simulink model "Control_software_v1_1"  (R2017a)
settings: Solver=FixedStepDiscrete  StartTime=0.0  StopTime=inf  FixedStep=Ts_main  RelTol=1e-3  EnableMultiTasking=on
InitFcn:
  | clc
  | eval('ContrPrm_v1_1')
model workspace (MAT data in the model file):
  JoyW_sat = 10
values from neighbouring files (symbols this model uses):
  Afilt_Winch = (Amatr_Winch-L_Winch*Cmatr_Winch)    [ContrPrm_v1_1.m]
  AOsat = 10    [ContrPrm_v1_1.m]
  Bfilt_Winch = [L_Winch Bmatr_Winch]    [ContrPrm_v1_1.m]
  Cfilt_Winch = eye(2)    [ContrPrm_v1_1.m]
  Dfilt_Winch = zeros(2)    [ContrPrm_v1_1.m]
  JoyS_gain = 5    [ContrPrm_v1_1.m]
  JoyS_ofst = -2.5    [ContrPrm_v1_1.m]
  JoyS_sat = 9.2    [ContrPrm_v1_1.m]
  JoyW_gain = -5    [ContrPrm_v1_1.m]
  JoyW_ofst = -2.5    [ContrPrm_v1_1.m]
  KspdWinch = 1    [ContrPrm_v1_1.m]
  NPotSpdEst = 3    [ContrPrm_v1_1.m]
  Pot_gain = PotMax/5    (= 0.08)    [ContrPrm_v1_1.m]
  Pot_max = PotMax    (= 0.4)    [ContrPrm_v1_1.m]
  Pot_min = 0    [ContrPrm_v1_1.m]
  Pot_ofst = -0.0558    [ContrPrm_v1_1.m]
  Ts_1ms = 1e-3    (= 0.001)    [ContrPrm_v1_1.m]
  Ts_1s = 1    [ContrPrm_v1_1.m]
  WinchDrumRad = 0.1    [ContrPrm_v1_1.m]
  WinchMotPosAIgain = WinchRevMax/WinchVoltMax*rev2rad    (= 76)    [ContrPrm_v1_1.m]
  WinchMotTorqueMax = 13    [ContrPrm_v1_1.m]
  WinchRefSpdSup = 15/WinchDrumRad    (= 150)    [ContrPrm_v1_1.m]
  WinchTravelMin_m = -2    [ContrPrm_v1_1.m]
  WinchVoltMax = 10    [ContrPrm_v1_1.m]
  x0_Winch = [0;0]    [ContrPrm_v1_1.m]
undefined symbols (not defined in the file or in its folder): C, datevec, JoyFiltDen, JoyFiltNum, PotPosFiltDen, PotPosFiltNum, WinchPosFiltDen, WinchPosFiltNum, WinchSpdEstFiltDen, WinchSpdEstFiltNum
libraries: xpcnilib x6, slrtlib x6, xpcseriallib x4, simulink x4, speedgoatlib_IO751 x3, etargetslib x2, xpcwalltimelib x1
(part 1 of 2)
settings Model: sg_rtwmakecfg_data=_sg_netxLib_MSVC140_  SimulationMode=external  Creator=Philip Hu  LastModifiedBy=admin
settings SolverCC: EnableConcurrentExecution=on
settings DataIOCC: SaveFormat=Array  SignalLoggingSaveFormat=ModelDataLogs  SaveOutput=off  SignalLogging=off  SaveTime=off
settings OptimizationCC: BlockReduction=off  OptimizeBlockIOStorage=off  BufferReuse=off  GlobalBufferReuse=off  ExpressionFolding=off  ExpressionDepthLimit=2147483647  LocalBlockOutputs=off  LifeSpan=inf
settings DebuggingCC: SolverPrmCheckMsg=warning  FcnCallInpInsideContextMsg=warning  StateNameClashWarn=warning  SFUnexpectedBacktrackingDiag=warning  SFNoUnconditionalDefaultTransitionDiag=warning  SFExecutionAtInitializationDiag=none
settings HardwareCC: ProdBitPerPointer=32  ProdBitPerSizeT=32  ProdBitPerPtrDiffT=32  ProdLargestAtomicFloat=None  ProdWordSize=32  ProdLongLongMode=on  ProdHWDeviceType=Generic->32-bit x86 compatible
settings ModelReferenceCC: PropagateSignalLabelsOutOfModel=off
settings SFSimCC: SimParseCustomCode=off
settings RTWCC: SystemTargetFile=slrt.tlc  TemplateMakefile=slrt_default_tmf  Description=Simulink Real-Time  RTWCompilerOptimization=on
settings SimulinkRealTimeCC: GeneratePreprocessorConditionals=Disable all  RL32ObjectName=AWE  xPCModelTimeoutSecs=20
settings ConfigComp: CovMetricSettings=dw  CovHtmlReporting=on  CovSaveCumulativeToWorkspaceVar=on  CovSaveSingleToWorkspaceVar=on  CovExternalEMLEnable=off  CovSFcnEnable=off

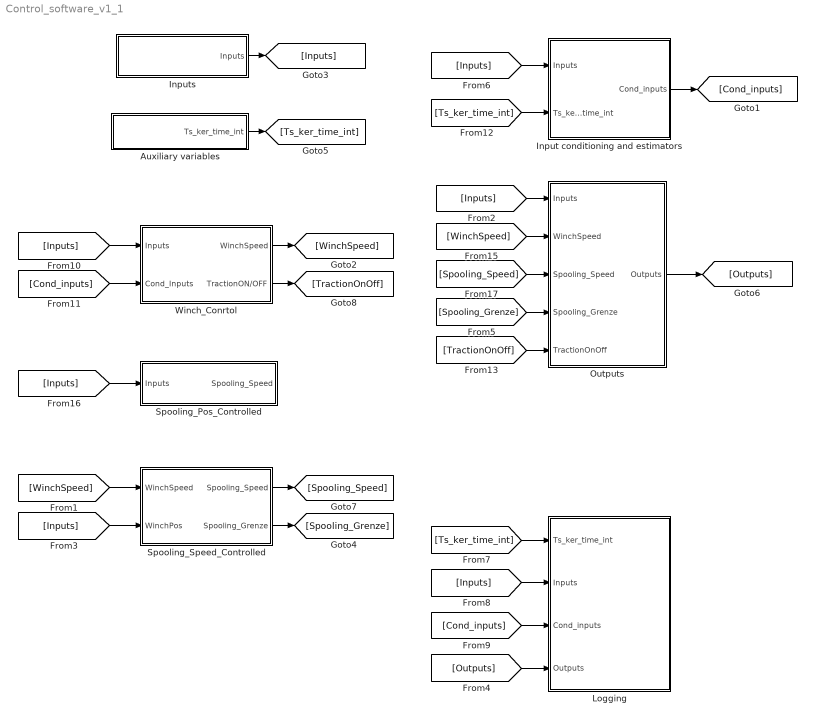
== system Control_software_v1_1 ==
  Auxiliary variables : Subsystem
  Input conditioning and estimators : Subsystem
  Inputs : Subsystem
  Logging : Subsystem
  Outputs : Subsystem
  Spooling_Pos_Controlled : Subsystem
  Spooling_Speed_Controlled : Subsystem
  Winch_Conrtol : Subsystem
  wires:
  Auxiliary variables/1(Ts_ker_time_int) -> [Ts_ker_time_int]
  [Ts_ker_time_int] -> Logging/1(Ts_ker_time_int)
  Outputs/1(Outputs) -> [Outputs]
  [Cond_inputs] -> Logging/3(Cond_inputs)
  Inputs/1(Inputs) -> [Inputs]
  Input conditioning and estimators/1(Cond_inputs) -> [Cond_inputs]
  [Outputs] -> Logging/4(Outputs)
  [Inputs] -> Input conditioning and estimators/1(Inputs)
  [Inputs] -> Logging/2(Inputs)
  [Ts_ker_time_int] -> Input conditioning and estimators/2(Ts_ker_time_int)
  [Inputs] -> Outputs/1(Inputs)
  [Inputs] -> Winch_Conrtol/1(Inputs)
  [Cond_inputs] -> Winch_Conrtol/2(Cond_Inputs)
  Winch_Conrtol/1(WinchSpeed) -> [WinchSpeed]
  [WinchSpeed] -> Outputs/2(WinchSpeed)
  [Inputs] -> Spooling_Pos_Controlled/1(Inputs)
  [Spooling_Speed] -> Outputs/3(Spooling_Speed)
  [WinchSpeed] -> Spooling_Speed_Controlled/1(WinchSpeed)
  [Inputs] -> Spooling_Speed_Controlled/2(WinchPos)
  Spooling_Speed_Controlled/1(Spooling_Speed) -> [Spooling_Speed]
  Spooling_Speed_Controlled/2(Spooling_Grenze) -> [Spooling_Grenze]
  [Spooling_Grenze] -> Outputs/4(Spooling_Grenze)
  Winch_Conrtol/2(TractionON/OFF) -> [TractionOnOff]
  [TractionOnOff] -> Outputs/5(TractionOnOff)

== system Control_software_v1_1/Auxiliary variables ==
  Constat : Constant  Value=Ts_1s  SampleTime=Ts_1s
  Sum : Sum  Inputs=|++
  Unit Delay : UnitDelay  SampleTime=-1
  Ts_ker_time_int : Outport
  wires:
  Constat/1 -> Sum/1
  Sum/1 -> Ts_ker_time_int/1, Unit Delay/1
  Unit Delay/1 -> Sum/2

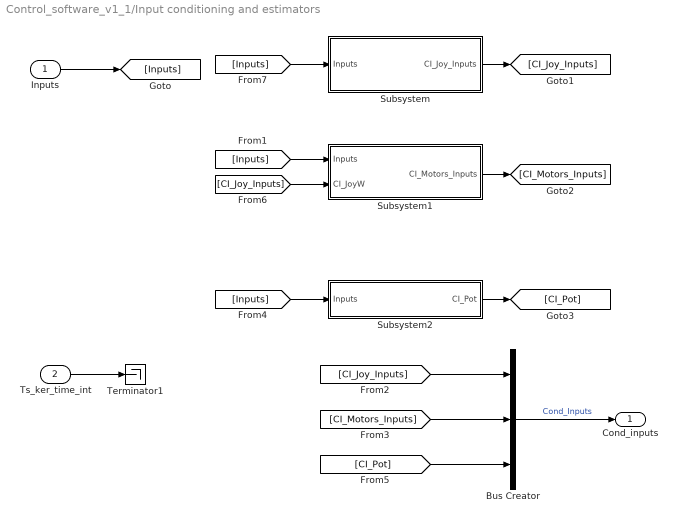
== system Control_software_v1_1/Input conditioning and estimators ==
  Inputs : Inport
  Ts_ker_time_int : Inport  Port=2
  Bus Creator : BusCreator  Inputs=3
  Subsystem : Subsystem
  Subsystem1 : Subsystem
  Subsystem2 : Subsystem
  Terminator1 : Terminator
  Cond_inputs : Outport
  wires:
  Inputs/1 -> [Inputs]
  Ts_ker_time_int/1 -> Terminator1/1
  [Inputs] -> Subsystem/1(Inputs)
  Subsystem/1(CI_Joy_Inputs) -> [CI_Joy_Inputs]
  Bus Creator/1 -> Cond_inputs/1  "Cond_Inputs"
  [Inputs] -> Subsystem1/1(Inputs)
  Subsystem1/1(CI_Motors_Inputs) -> [CI_Motors_Inputs]
  [Inputs] -> Subsystem2/1(Inputs)
  Subsystem2/1(CI_Pot) -> [CI_Pot]
  [CI_Pot] -> Bus Creator/3
  [CI_Motors_Inputs] -> Bus Creator/2
  [CI_Joy_Inputs] -> Bus Creator/1
  [CI_Joy_Inputs] -> Subsystem1/2(CI_JoyW)

== system Control_software_v1_1/Inputs ==
  Analog Inputs : Subsystem
  Bus Creator2 : BusCreator  Inputs=5
  Digital Inputs : Subsystem
  RS232_read : Subsystem
  Inputs : Outport
  wires:
  Analog Inputs/1(Analog_inputs) -> Bus Creator2/1
  Digital Inputs/1(DgInputs) -> Bus Creator2/2
  Bus Creator2/1 -> Inputs/1
  RS232_read/2(GPS_data) -> Bus Creator2/4
  RS232_read/1(IMU_data) -> Bus Creator2/3
  RS232_read/3(GU_Yaw) -> Bus Creator2/5

== system Control_software_v1_1/Logging ==
  Ts_ker_time_int : Inport
  Inputs : Inport  Port=2
  Cond_inputs : Inport  Port=3
  Outputs : Inport  Port=4
  Bus Creator1 : BusCreator  Inputs=2
  Data Type Conversion1 : DataTypeConversion  OutDataTypeStr=double
  Log_conditioning : Subsystem
  MavLink_log : slrtlib/Displays and Logging/Scope   scopeno=1  scopetype=File  autostart=on  viewmode=Graphical redraw  formatstr='%15.6f'  grid=on  ylimits=[0,0]  nosamples=1000  noprepostsamples=0  interleave=1  triggermode=FreeRun  triggersignal=1  trigsignalfromport=off  triggerlevel=0.0  triggerslope=Either  triggerscope=1  triggersample=0  filename=Var_MVLK.dat  mode=Lazy  writesize=512  autorestart=on  dynamicfilemode=off  maxwritefilesize=512*1024^2
  TS100_log : slrtlib/Displays and Logging/Scope   scopeno=3  scopetype=File  autostart=on  viewmode=Graphical redraw  formatstr='%15.6f'  grid=on  ylimits=[0,0]  nosamples=1000  noprepostsamples=0  interleave=1  triggermode=FreeRun  triggersignal=1  trigsignalfromport=off  triggerlevel=0.0  triggerslope=Either  triggerscope=1  triggersample=0  filename=Var_100.dat  mode=Commit  writesize=512  autorestart=on  dynamicfilemode=off  maxwritefilesize=512*1024^2
  TS1_log : slrtlib/Displays and Logging/Scope   scopeno=2  scopetype=File  autostart=on  viewmode=Graphical redraw  formatstr='%15.6f'  grid=on  ylimits=[0,0]  nosamples=1000  noprepostsamples=0  interleave=1  triggermode=FreeRun  triggersignal=1  trigsignalfromport=off  triggerlevel=0.0  triggerslope=Either  triggerscope=1  triggersample=0  filename=Var_1.dat  mode=Commit  writesize=512  autorestart=on  dynamicfilemode=off  maxwritefilesize=512*1024^2
  Time_Scope_trigger : Subsystem
  Time_log : slrtlib/Displays and Logging/Scope   scopeno=4  scopetype=File  autostart=on  viewmode=Graphical sliding  formatstr='%15.6f'  grid=off  ylimits=[0,0]  nosamples=10  noprepostsamples=0  interleave=1  triggermode=Signal triggering  triggersignal=2  trigsignalfromport=off  triggerlevel=0.5  triggerslope=Either  triggerscope=1  triggersample=0  filename=Var_Time.dat  mode=Commit  writesize=512  autorestart=off  dynamicfilemode=off  maxwritefilesize=512*1024^2
  Wall Time 1 : xpcwalltimelib/Wall Time   TimeFormat=Date  EpochSource=MATLAB  EpochVector=datevec('01/01/1970')  InputTrigger=off  SampleTime=Ts_1s
  wires:
  Log_conditioning/2(T100_log) -> TS100_log/1
  Bus Creator1/1 -> Time_log/1  "Date_time"
  Time_Scope_trigger/1(Trigger_time) -> Bus Creator1/2
  Ts_ker_time_int/1 -> Time_Scope_trigger/1(In1)
  Outputs/1 -> Log_conditioning/3(Outputs)
  Cond_inputs/1 -> Log_conditioning/2(Cond_inputs)
  Inputs/1 -> Log_conditioning/1(Inputs)
  Log_conditioning/1(MaVLink_log) -> MavLink_log/1
  Log_conditioning/3(T1_log) -> TS1_log/1
  Wall Time 1/1 -> Data Type Conversion1/1
  Data Type Conversion1/1 -> Bus Creator1/1

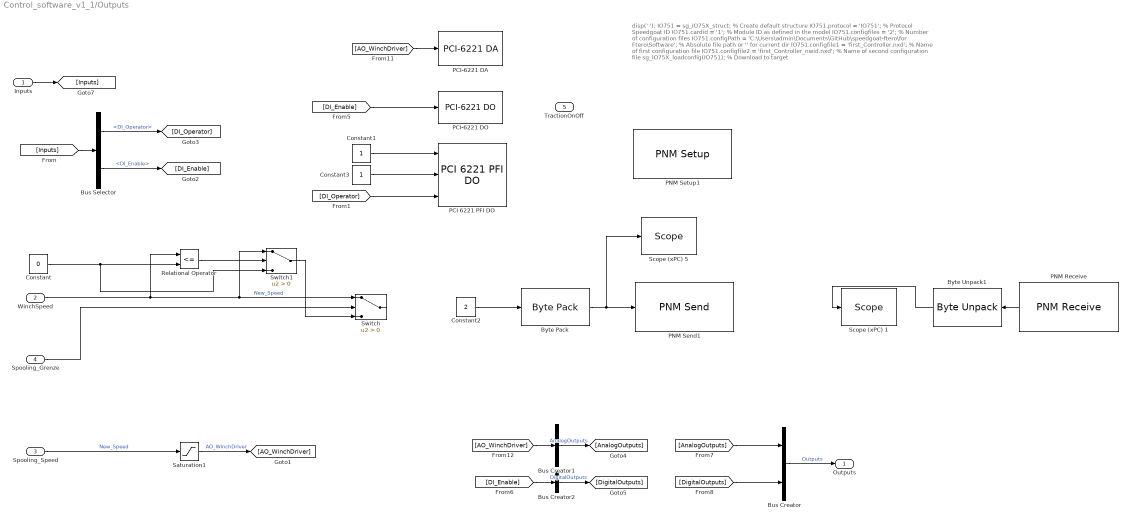
== system Control_software_v1_1/Outputs ==
  note: disp(' ');
      |     IO751 = sg_IO75X_struct;				 											% Create default structure
      |
      |     IO751.protocol = 'IO751';				 											% Protocol Speedgoat ID
      |     IO751.cardid = '1';						 											% Module ID as defined in the model
      |     IO751.configfiles = '2';					 											% Number of configuration files
      |     IO751.configPath = 'C:\Users\admin\Documents\GitHub\speedgoat-ftero\for Ftero\Software';	 % Absolute file path or '' for current dir
      |     IO751.configfile1 = 'first_Controller.nxd';	 											% Name of first configuration file
      |     IO751.configfile2 = 'first_Controller_nwid.nxd'; 											% Name of second configuration file
      |
      |     sg_IO75X_loadconfig(IO751);														% Download to target
  Inputs : Inport
  WinchSpeed : Inport  Port=2
  Spooling_Speed : Inport  Port=3
  Spooling_Grenze : Inport  Port=4
  TractionOnOff : Inport  Port=5
  Bus Creator : BusCreator  Inputs=2
  Bus Creator1 : BusCreator  Inputs=1
  Bus Creator2 : BusCreator  Inputs=1
  Bus Selector : BusSelector  OutputSignals=DgInputs.DI_Operator,DgInputs.DI_Enable
  Byte Pack : etargetslib/Byte Pack  datatypes={'uint8'}  byteAlign=1
  Byte Unpack1 : etargetslib/Byte Unpack  dimensions={1}  datatypes={'uint8'}  byteAlign=1
  Constant : Constant  Value=0
  Constant1 : Constant
  Constant2 : Constant  Value=2  OutDataTypeStr=uint8
  Constant3 : Constant
  "PCI 6221 PFI DO " : xpcnilib/Digital Output/M Series/PCI 6221 PFI DO   channel=[0 2 3]  reset=[0]  initial=[1 1 0]  sampleTime=Ts_1ms  slot=-1
      settings: SourceProductName=Simulink Real-Time  SourceProductBaseCode=XP
  PCI-6221 DA : xpcnilib/D//A/M Series/PCI-6221 DA  channel=[2]  reset=[1]  initValue=[0]  sampletime=Ts_1ms  slot=-1
      settings: SourceProductName=Simulink Real-Time  SourceProductBaseCode=XP
  PCI-6221 DO : xpcnilib/Digital Output/M Series/PCI-6221 DO  channel=[6]  reset=[0]  initValue=[0]  sampletime=Ts_1ms  slot=-1
      settings: SourceProductName=Simulink Real-Time  SourceProductBaseCode=XP
  PNM Receive : speedgoatlib_IO751/PNM Receive  id=1  portType=1 port with n element vector of type UINT8  inputOutput=1  sampleTime=0.001
  PNM Send1 : speedgoatlib_IO751/PNM Send  id=1  portType=1 port with n element vector of type UINT8  inputOutput=1  sampleTime=0.001
  PNM Setup1 : speedgoatlib_IO751/PNM Setup  id=1  driveLetter=C:  configurationMode=Configuration file  mode=Polling mode  sampleTime=0.001  pciSlot=-1  quantityOfAcyclicObjects=0
  Relational Operator : RelationalOperator  Operator=<=  OutDataTypeStr=boolean  RndMeth=Simplest
  Saturation1 : Saturate  UpperLimit=AOsat  LowerLimit=-AOsat
  Scope (xPC) 1 : slrtlib/Displays and Logging/Scope   scopeno=7  scopetype=Target  autostart=on  viewmode=Numerical  formatstr='%15.6f'  grid=on  ylimits=[0,0]  nosamples=3  noprepostsamples=0  interleave=1  triggermode=FreeRun  triggersignal=1  trigsignalfromport=off  triggerlevel=0.0  triggerslope=Either  triggerscope=1  triggersample=0  filename=data.dat  mode=Lazy  writesize=512  autorestart=off  dynamicfilemode=off  maxwritefilesize=512*1024^2
  Scope (xPC) 5 : slrtlib/Displays and Logging/Scope   scopeno=5  scopetype=Target  autostart=on  viewmode=Numerical  formatstr='%15.6f'  grid=on  ylimits=[0,0]  nosamples=3  noprepostsamples=0  interleave=1  triggermode=FreeRun  triggersignal=1  trigsignalfromport=off  triggerlevel=0.0  triggerslope=Either  triggerscope=1  triggersample=0  filename=data.dat  mode=Lazy  writesize=512  autorestart=off  dynamicfilemode=off  maxwritefilesize=512*1024^2
  Switch : Switch  Criteria=u2 > Threshold  OutDataTypeStr=uint8
  Switch1 : Switch  Criteria=u2 > Threshold
  Outputs : Outport
  wires:
  Inputs/1 -> [Inputs]
  [Inputs] -> Bus Selector/1
  Bus Creator/1 -> Outputs/1  "Outputs"
  [AnalogOutputs] -> Bus Creator/1
  [DigitalOutputs] -> Bus Creator/2
  Bus Selector/1 -> [DI_Operator]  "<DI_Operator>"
  Bus Creator1/1 -> [AnalogOutputs]  "AnalogOutputs"
  Bus Creator2/1 -> [DigitalOutputs]  "DigitalOutputs"
  Constant3/1 -> "PCI 6221 PFI DO "/2
  [AO_WinchDriver] -> PCI-6221 DA/1
  [AO_WinchDriver] -> Bus Creator1/1
  [DI_Enable] -> Bus Creator2/1
  [DI_Enable] -> PCI-6221 DO/1
  Bus Selector/2 -> [DI_Enable]  "<DI_Enable>"
  [DI_Operator] -> "PCI 6221 PFI DO "/3
  Constant1/1 -> "PCI 6221 PFI DO "/1
  Spooling_Speed/1 -> Saturation1/1  "New_Speed"
  WinchSpeed/1 -> Relational Operator/1, Switch1/1, Switch/1  "New_Speed"
  Spooling_Grenze/1 -> Switch/2
  Constant/1 -> Switch1/3, Relational Operator/2
  Relational Operator/1 -> Switch1/2
  Switch1/1 -> Switch/3
  Saturation1/1 -> [AO_WinchDriver]  "AO_WinchDriver"
  Byte Pack/1 -> Scope (xPC) 5/1, PNM Send1/1
  PNM Receive/1 -> Byte Unpack1/1
  Byte Unpack1/1 -> Scope (xPC) 1/1
  Constant2/1 -> Byte Pack/1

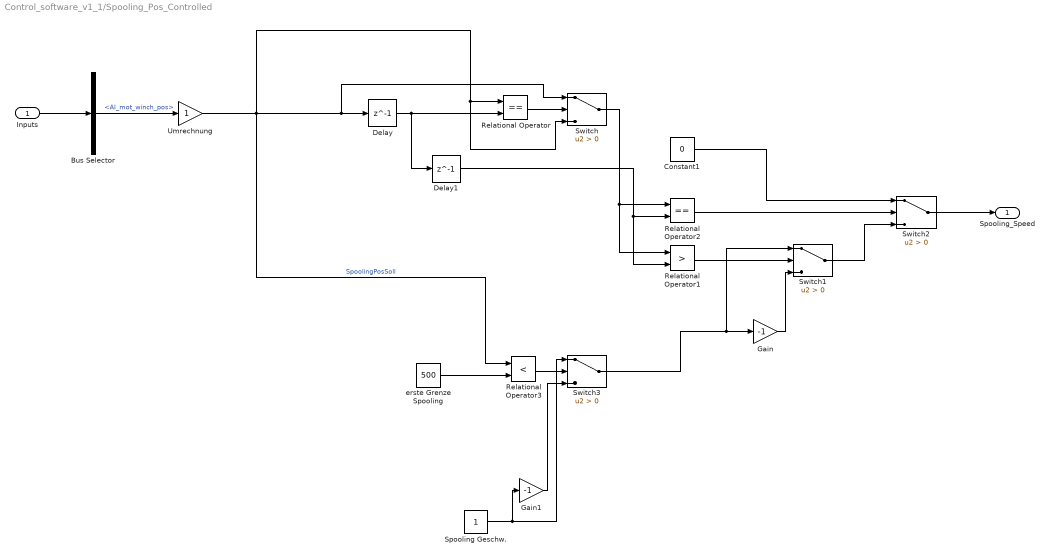
== system Control_software_v1_1/Spooling_Pos_Controlled ==
  Inputs : Inport
  Bus Selector : BusSelector  OutputSignals=Analog_inputs.AI_mot_winch_pos
  Constant1 : Constant  Value=0
  Delay : Delay  DelayLength=1  InitialCondition=0
  Delay1 : Delay  DelayLength=1  InitialCondition=0
  Gain : Gain  Gain=-1
  Gain1 : Gain  Gain=-1
  Relational Operator : RelationalOperator  Operator===  OutDataTypeStr=boolean  RndMeth=Simplest
  Relational Operator1 : RelationalOperator  Operator=>  OutDataTypeStr=boolean  RndMeth=Simplest
  Relational Operator2 : RelationalOperator  Operator===  OutDataTypeStr=boolean  RndMeth=Simplest
  Relational Operator3 : RelationalOperator  Operator=<  OutDataTypeStr=boolean  RndMeth=Simplest
  Spooling Geschw. : Constant
  Switch{,1..3} (4 alike) : Switch  Criteria=u2 > Threshold
  Umrechnung : Gain
  erste Grenze Spooling : Constant  Value=500
  Spooling_Speed : Outport
  wires:
  Inputs/1 -> Bus Selector/1
  Bus Selector/1 -> Umrechnung/1  "<AI_mot_winch_pos>"
  Umrechnung/1 -> Switch/3, Relational Operator/1, Relational Operator3/1, Switch/1, Delay/1  "SpoolingPosSoll"
  Relational Operator/1 -> Switch/2
  Switch/1 -> Relational Operator2/1, Relational Operator1/1
  Delay/1 -> Delay1/1, Relational Operator/2
  Relational Operator1/1 -> Switch1/2
  Constant1/1 -> Switch2/1
  Relational Operator2/1 -> Switch2/2
  Delay1/1 -> Relational Operator2/2, Relational Operator1/2
  Switch1/1 -> Switch2/3
  Gain/1 -> Switch1/3
  Relational Operator3/1 -> Switch3/2
  erste Grenze Spooling/1 -> Relational Operator3/2
  Switch3/1 -> Switch1/1, Gain/1
  Spooling Geschw./1 -> Gain1/1, Switch3/1
  Gain1/1 -> Switch3/3
  Switch2/1 -> Spooling_Speed/1

== system Control_software_v1_1/Spooling_Speed_Controlled ==
  WinchSpeed : Inport
  WinchPos : Inport  Port=2
  Bus Selector : BusSelector  OutputSignals=Analog_inputs.AI_mot_winch_pos
  Gain : Gain  Gain=-1
  Gain1 : Gain  Gain=2
  Relational Operator : RelationalOperator  Operator=<  OutDataTypeStr=boolean  RndMeth=Simplest
  Relational Operator1 : RelationalOperator  Operator=<  OutDataTypeStr=boolean  RndMeth=Simplest
  Spooling Grenze : Constant  Value=500
  Switch : Switch  Criteria=u2 > Threshold
  Umrechnung : Gain  Gain=0.01
  Umrechnung1 : Gain  Gain=0.1
  Spooling_Speed : Outport
  Spooling_Grenze : Outport  Port=2
  wires:
  WinchPos/1 -> Bus Selector/1
  Bus Selector/1 -> Umrechnung/1  "<AI_mot_winch_pos>"
  WinchSpeed/1 -> Umrechnung1/1
  Umrechnung/1 -> Relational Operator1/1, Relational Operator/1  "SpoolingPosSoll"
  Spooling Grenze/1 -> Gain1/1, Relational Operator/2
  Umrechnung1/1 -> Gain/1, Switch/1
  Gain/1 -> Switch/3
  Gain1/1 -> Relational Operator1/2
  Relational Operator/1 -> Switch/2
  Relational Operator1/1 -> Spooling_Grenze/1
  Switch/1 -> Spooling_Speed/1

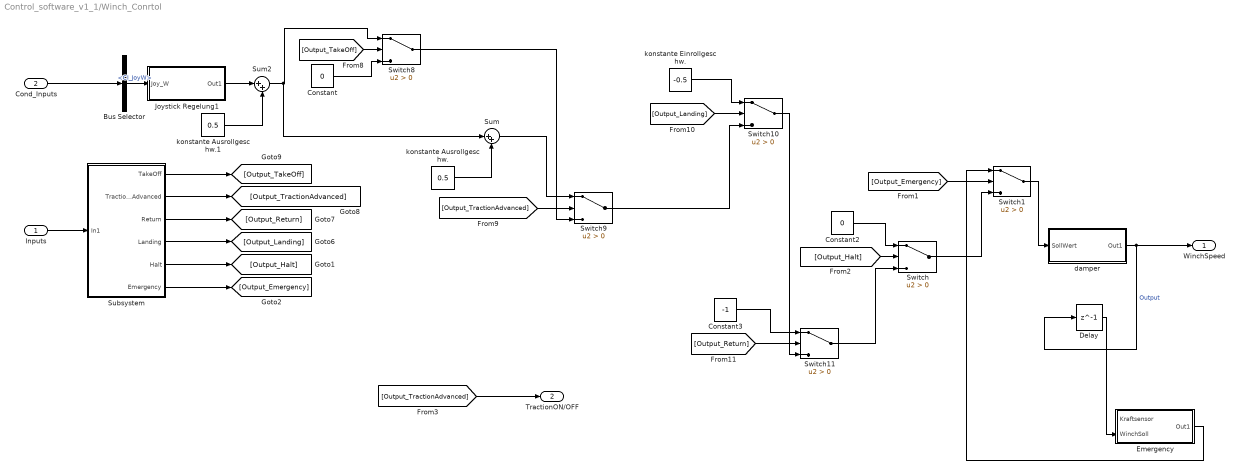
== system Control_software_v1_1/Winch_Conrtol ==
  Inputs : Inport
  Cond_Inputs : Inport  Port=2
  Bus Selector : BusSelector  OutputSignals=CI_Joy_Inputs.CI_JoyW
  Constant : Constant  Value=0
  Constant2 : Constant  Value=0
  Constant3 : Constant  Value=-1
  Delay : Delay  DelayLength=1  InitialCondition=0
  Emergency : Subsystem
  Joystick Regelung1 : Subsystem
  Subsystem : Subsystem
  Sum : Sum  Inputs=|++
  Sum2 : Sum  Inputs=|++
  Switch{,1,8..11} (6 alike) : Switch  Criteria=u2 > Threshold
  damper : Subsystem
  konstante Ausrollgeschw. : Constant  Value=0.5
  konstante Ausrollgeschw.1 : Constant  Value=0.5
  konstante Einrollgeschw. : Constant  Value=-0.5
  WinchSpeed : Outport
  TractionON/OFF : Outport  Port=2
  wires:
  Inputs/1 -> Subsystem/1(In1)
  [Output_TakeOff] -> Switch8/2
  [Output_TractionAdvanced] -> Switch9/2
  konstante Einrollgeschw./1 -> Switch10/1
  Switch10/1 -> Switch11/3
  [Output_Return] -> Switch11/2
  Subsystem/1(TakeOff) -> [Output_TakeOff]
  Subsystem/2(TractionAdvanced) -> [Output_TractionAdvanced]
  Subsystem/3(Return) -> [Output_Return]
  Subsystem/4(Landing) -> [Output_Landing]
  [Output_Landing] -> Switch10/2
  damper/1(Out1) -> WinchSpeed/1, Delay/1  "Output"
  Constant/1 -> Switch8/3
  Cond_Inputs/1 -> Bus Selector/1
  [Output_Halt] -> Switch/2
  [Output_Emergency] -> Switch1/2
  Constant2/1 -> Switch/1
  Switch11/1 -> Switch/3
  Switch/1 -> Switch1/3
  Delay/1 -> Emergency/2(WinchSoll)
  Emergency/1(Out1) -> Switch1/1
  Switch1/1 -> damper/1(SollWert)
  ? -> Emergency/1(Kraftsensor)
  Constant3/1 -> Switch11/1
  Subsystem/6(Emergency) -> [Output_Emergency]
  Subsystem/5(Halt) -> [Output_Halt]
  Switch8/1 -> Switch9/3
  Switch9/1 -> Switch10/3
  konstante Ausrollgeschw.1/1 -> Sum2/2
  Joystick Regelung1/1(Out1) -> Sum2/1
  Bus Selector/1 -> Joystick Regelung1/1(Joy_W)  "<CI_JoyW>"
  konstante Ausrollgeschw./1 -> Sum/2
  Sum2/1 -> Sum/1, Switch8/1
  Sum/1 -> Switch9/1
  [Output_TractionAdvanced] -> TractionON/OFF/1

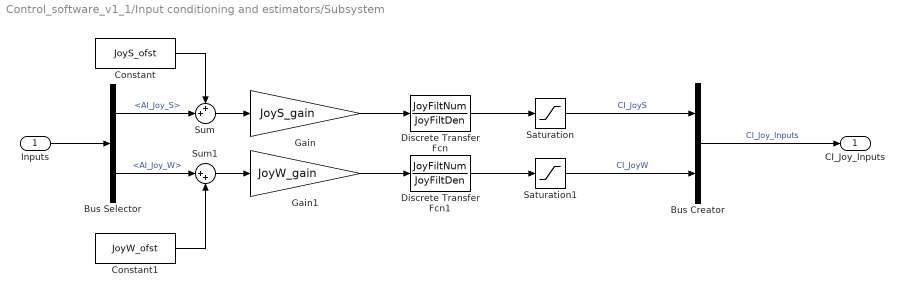
== system Control_software_v1_1/Input conditioning and estimators/Subsystem ==
  Inputs : Inport
  Bus Creator : BusCreator  Inputs=2
  Bus Selector : BusSelector  OutputSignals=Analog_inputs.AI_Joy_S,Analog_inputs.AI_Joy_W
  Constant : Constant  Value=JoyS_ofst
  Constant1 : Constant  Value=JoyW_ofst
  Discrete Transfer Fcn : DiscreteTransferFcn  Numerator=JoyFiltNum  Denominator=JoyFiltDen
  Discrete Transfer Fcn1 : DiscreteTransferFcn  Numerator=JoyFiltNum  Denominator=JoyFiltDen
  Gain : Gain  Gain=JoyS_gain
  Gain1 : Gain  Gain=JoyW_gain
  Saturation : Saturate  UpperLimit=JoyS_sat  LowerLimit=-JoyS_sat
  Saturation1 : Saturate  UpperLimit=JoyW_sat  LowerLimit=-JoyW_sat
  Sum : Sum  Inputs=++|
  Sum1 : Sum  Inputs=|++
  CI_Joy_Inputs : Outport
  wires:
  Discrete Transfer Fcn/1 -> Saturation/1
  Saturation/1 -> Bus Creator/1  "CI_JoyS"
  Sum1/1 -> Gain1/1
  Constant/1 -> Sum/1
  Inputs/1 -> Bus Selector/1
  Discrete Transfer Fcn1/1 -> Saturation1/1
  Gain/1 -> Discrete Transfer Fcn/1
  Bus Selector/1 -> Sum/2  "<AI_Joy_S>"
  Saturation1/1 -> Bus Creator/2  "CI_JoyW"
  Bus Selector/2 -> Sum1/1  "<AI_Joy_W>"
  Bus Creator/1 -> CI_Joy_Inputs/1  "CI_Joy_Inputs"
  Gain1/1 -> Discrete Transfer Fcn1/1
  Constant1/1 -> Sum1/2
  Sum/1 -> Gain/1

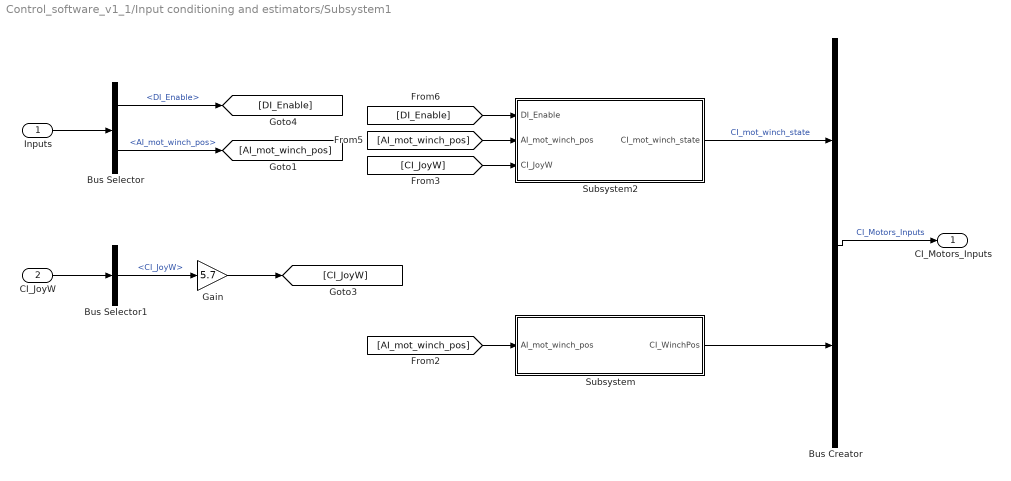
== system Control_software_v1_1/Input conditioning and estimators/Subsystem1 ==
  Inputs : Inport
  CI_JoyW : Inport  Port=2
  Bus Creator : BusCreator  Inputs=2
  Bus Selector : BusSelector  OutputSignals=DgInputs.DI_Enable,Analog_inputs.AI_mot_winch_pos
  Bus Selector1 : BusSelector  OutputSignals=CI_JoyW
  Gain : Gain  Gain=5.7
  Subsystem : Subsystem
  Subsystem2 : Subsystem
  CI_Motors_Inputs : Outport
  wires:
  Bus Selector/2 -> [AI_mot_winch_pos]  "<AI_mot_winch_pos>"
  Bus Creator/1 -> CI_Motors_Inputs/1  "CI_Motors_Inputs"
  Inputs/1 -> Bus Selector/1
  Subsystem2/1(CI_mot_winch_state) -> Bus Creator/1  "CI_mot_winch_state"
  [CI_JoyW] -> Subsystem2/3(CI_JoyW)
  [AI_mot_winch_pos] -> Subsystem2/2(AI_mot_winch_pos)
  [AI_mot_winch_pos] -> Subsystem/1(AI_mot_winch_pos)
  Subsystem/1(CI_WinchPos) -> Bus Creator/2
  CI_JoyW/1 -> Bus Selector1/1
  Bus Selector1/1 -> Gain/1  "<CI_JoyW>"
  Bus Selector/1 -> [DI_Enable]  "<DI_Enable>"
  [DI_Enable] -> Subsystem2/1(DI_Enable)
  Gain/1 -> [CI_JoyW]

== system Control_software_v1_1/Input conditioning and estimators/Subsystem2 ==
  Inputs : Inport
  Bus Creator : BusCreator  Inputs=2
  Bus Selector : BusSelector  OutputSignals=Analog_inputs.AI_pot_pos
  Constant : Constant  Value=Pot_ofst
  Delay : Delay  DelayLength=NPotSpdEst
  Discrete Transfer Fcn1 : DiscreteTransferFcn  Numerator=PotPosFiltNum  Denominator=PotPosFiltDen
  Gain : Gain  Gain=Pot_gain
  Gain1 : Gain  Gain=1/(NPotSpdEst*Ts_1ms)
  Saturation : Saturate  UpperLimit=Pot_max  LowerLimit=Pot_min
  Sum : Sum  Inputs=++|
  Sum1 : Sum  Inputs=+-|
  CI_Pot : Outport
  wires:
  Inputs/1 -> Bus Selector/1
  Bus Creator/1 -> CI_Pot/1  "CI_Pot"
  Discrete Transfer Fcn1/1 -> Saturation/1
  Constant/1 -> Sum/1
  Bus Selector/1 -> Gain/1  "<AI_pot_pos>"
  Sum/1 -> Discrete Transfer Fcn1/1
  Gain/1 -> Sum/2
  Saturation/1 -> [CI_PotPos], Bus Creator/1  "CI_PotPos"
  Delay/1 -> Sum1/2
  Sum1/1 -> Gain1/1
  Gain1/1 -> Bus Creator/2  "CI_PotSpd"
  [CI_PotPos] -> Sum1/1, Delay/1

== system Control_software_v1_1/Inputs/Analog Inputs ==
  Bus Creator : BusCreator  Inputs=5
  PCI-6221 AD : xpcnilib/A//D/M Series/PCI-6221 AD  channel=[1 2 4 5 6]  range=[5 5 10 10 5]  coupling=[0 0 2 2 0]  scantime=5e-6  sampletime=Ts_1ms  slot=-1
      settings: SourceProductName=Simulink Real-Time  SourceProductBaseCode=XP
  Analog_inputs : Outport
  wires:
  Bus Creator/1 -> Analog_inputs/1  "Analog_inputs"
  PCI-6221 AD/1 -> Bus Creator/1  "AI_Joy_W"
  PCI-6221 AD/2 -> Bus Creator/2  "AI_Joy_S"
  PCI-6221 AD/3 -> Bus Creator/3  "AI_mot_slide_pos"
  PCI-6221 AD/4 -> Bus Creator/4  "AI_mot_winch_pos"
  PCI-6221 AD/5 -> Bus Creator/5  "AI_pot_pos"

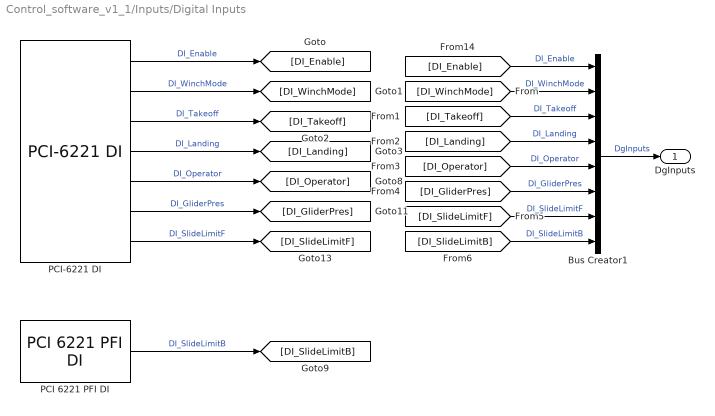
== system Control_software_v1_1/Inputs/Digital Inputs ==
  Bus Creator1 : BusCreator  Inputs=8
  "PCI 6221 PFI DI " : xpcnilib/Digital Input/M Series/PCI 6221 PFI DI   channel=[1]  sampleTime=Ts_1ms  slot=-1
      settings: SourceProductName=Simulink Real-Time  SourceProductBaseCode=XP
  PCI-6221 DI : xpcnilib/Digital Input/M Series/PCI-6221 DI  channel=[1 2 3 4 5 7 8]  sampletime=Ts_1ms  slot=-1
      settings: SourceProductName=Simulink Real-Time  SourceProductBaseCode=XP
  DgInputs : Outport
  wires:
  Bus Creator1/1 -> DgInputs/1  "DgInputs"
  [DI_Enable] -> Bus Creator1/1  "DI_Enable"
  [DI_WinchMode] -> Bus Creator1/2  "DI_WinchMode"
  [DI_Takeoff] -> Bus Creator1/3  "DI_Takeoff"
  [DI_Landing] -> Bus Creator1/4  "DI_Landing"
  [DI_Operator] -> Bus Creator1/5  "DI_Operator"
  [DI_GliderPres] -> Bus Creator1/6  "DI_GliderPres"
  [DI_SlideLimitF] -> Bus Creator1/7  "DI_SlideLimitF"
  [DI_SlideLimitB] -> Bus Creator1/8  "DI_SlideLimitB"
  PCI-6221 DI/1 -> [DI_Enable]  "DI_Enable"
  PCI-6221 DI/2 -> [DI_WinchMode]  "DI_WinchMode"
  PCI-6221 DI/3 -> [DI_Takeoff]  "DI_Takeoff"
  PCI-6221 DI/4 -> [DI_Landing]  "DI_Landing"
  PCI-6221 DI/5 -> [DI_Operator]  "DI_Operator"
  "PCI 6221 PFI DI "/1 -> [DI_SlideLimitB]  "DI_SlideLimitB"
  PCI-6221 DI/6 -> [DI_GliderPres]  "DI_GliderPres"
  PCI-6221 DI/7 -> [DI_SlideLimitF]  "DI_SlideLimitF"

== system Control_software_v1_1/Inputs/RS232_read ==
  Compass_read : Subsystem
  Constant{,1..3} (4 alike) : Constant  Value=0  OutDataTypeStr=Inherit: Inherit via back propagation  SampleTime=Ts_1s
  GPS_read : Subsystem
  IMU_read : Subsystem
  QSC-100 F : xpcseriallib/Quatech/QSC-100/QSC-100 F  group=FIFO Setup  port=2  irqnum=7  slot=-1  baud1=115200  parity1=None  ndata1=8  nstop1=1  fifomode1=64 deep  rlevel1=1  automode1=off  xmtfifosize1=1  xmtdatatype1=8 bit uint null terminated  rcvfifosize1=1024  baud2=4800  parity2=None  ndata2=8  nstop2=1  fifomode2=64 deep  rlevel2=1  automode2=off  xmtfifosize2=1  xmtdatatype2=8 bit uint null terminated  rcvfifosize2=512  baud3=57600  parity3=None  ndata3=8  nstop3=1  fifomode3=64 deep  rlevel3=1  automode3=off  xmtfifosize3=1  xmtdatatype3=8 bit uint null terminated  rcvfifosize3=1024  buad4=57600  parity4=None  ndata4=8  nstop4=1  fifomode4=64 deep  rlevel4=1  automode4=off  xmtfifosize4=1024  xmtdatatype4=8 bit uint null terminated  rcvfifosize4=1024
      settings: SourceProductName=Simulink Real-Time  SourceProductBaseCode=XP
  Terminator : Terminator
  IMU_data : Outport
  GPS_data : Outport  Port=2
  GU_Yaw : Outport  Port=3
  wires:
  Constant/1 -> QSC-100 F/1
  Constant1/1 -> QSC-100 F/2
  Constant2/1 -> QSC-100 F/3
  Constant3/1 -> QSC-100 F/4
  QSC-100 F/1 -> IMU_read/1(ASCII_IMU)
  QSC-100 F/2 -> GPS_read/1(ASCII_IMU)
  QSC-100 F/3 -> Compass_read/1(ASCII_IMU)
  IMU_read/1(IMU_data_valid) -> IMU_data/1
  GPS_read/1(GU_pos_data) -> GPS_data/1
  Compass_read/1(GU_Yaw) -> GU_Yaw/1
  QSC-100 F/4 -> Terminator/1

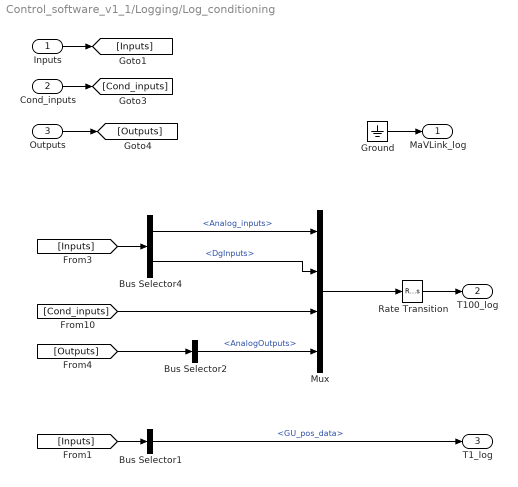
== system Control_software_v1_1/Logging/Log_conditioning ==
  Inputs : Inport
  Cond_inputs : Inport  Port=2
  Outputs : Inport  Port=3
  Bus Selector1 : BusSelector  OutputSignals=GU_pos_data
  Bus Selector2 : BusSelector  OutputSignals=AnalogOutputs
  Bus Selector4 : BusSelector  OutputSignals=Analog_inputs,DgInputs
  Ground : Ground
  Mux : Mux
  Rate Transition : RateTransition  OutPortSampleTime=Ts_10ms
  MaVLink_log : Outport
  T100_log : Outport  Port=2
  T1_log : Outport  Port=3
  wires:
  Cond_inputs/1 -> [Cond_inputs]
  Inputs/1 -> [Inputs]
  Outputs/1 -> [Outputs]
  [Inputs] -> Bus Selector4/1
  Ground/1 -> MaVLink_log/1
  Rate Transition/1 -> T100_log/1
  Bus Selector1/1 -> T1_log/1  "<GU_pos_data>"
  [Outputs] -> Bus Selector2/1
  Mux/1 -> Rate Transition/1
  Bus Selector4/1 -> Mux/1  "<Analog_inputs>"
  Bus Selector4/2 -> Mux/2  "<DgInputs>"
  [Cond_inputs] -> Mux/3
  [Inputs] -> Bus Selector1/1
  Bus Selector2/1 -> Mux/4  "<AnalogOutputs>"

== system Control_software_v1_1/Logging/Time_Scope_trigger ==
  In1 : Inport
  Constant : Constant  SampleTime=Ts_1s
  Constant1 : Constant  Value=0  SampleTime=Ts_1s
  Constant2 : Constant  Value=0  SampleTime=Ts_1s
  Switch : Switch  Threshold=2*Ts_1s
  Switch1 : Switch  Threshold=12*Ts_1s
  Trigger_time : Outport
  wires:
  In1/1 -> Switch/2, Switch1/2
  Constant/1 -> Switch/1
  Constant1/1 -> Switch/3
  Switch/1 -> Switch1/3
  Constant2/1 -> Switch1/1
  Switch1/1 -> Trigger_time/1  "Trigger_time"

== system Control_software_v1_1/Winch_Conrtol/Emergency ==
  Kraftsensor : Inport
  WinchSoll : Inport  Port=2
  Beschleunigung : Constant  Value=0.00125  SampleTime=0.001
  Gain : Gain  Gain=-1
  Relational Operator : RelationalOperator  OutDataTypeStr=boolean  RndMeth=Simplest
  Relational Operator1 : RelationalOperator  Operator=<  OutDataTypeStr=boolean  RndMeth=Simplest
  Sum : Sum  Inputs=|++
  Sum1 : Sum  Inputs=|++
  Switch : Switch  Criteria=u2 > Threshold
  Switch1 : Switch  Criteria=u2 > Threshold
  obere Kraftsensor Grenze : Constant  SampleTime=0.001
  untere Kraftsensor Grenze : Constant  Value=-1  SampleTime=0.001
  Out1 : Outport
  wires:
  obere Kraftsensor Grenze/1 -> Relational Operator/2
  Switch1/1 -> Out1/1
  Relational Operator/1 -> Switch/2
  WinchSoll/1 -> Sum1/2, Switch/3, Sum/2
  Kraftsensor/1 -> Relational Operator/1, Relational Operator1/1
  untere Kraftsensor Grenze/1 -> Relational Operator1/2
  Sum/1 -> Switch/1
  Sum1/1 -> Switch1/1
  Switch/1 -> Switch1/3
  Beschleunigung/1 -> Gain/1, Sum/1
  Gain/1 -> Sum1/1
  Relational Operator1/1 -> Switch1/2

== system Control_software_v1_1/Winch_Conrtol/Joystick Regelung1 ==
  Joy_W : Inport
  Delay : Delay  DelayLength=1  InitialCondition=0
  Joystick-Steuerung : Subsystem
  damper : Subsystem
  Out1 : Outport
  wires:
  Joy_W/1 -> Joystick-Steuerung/1(Joystick-Wert)
  Delay/1 -> Joystick-Steuerung/2(WinchSoll)
  damper/1(Out1) -> Delay/1, Out1/1
  Joystick-Steuerung/1(Out1) -> damper/1(SollWert)

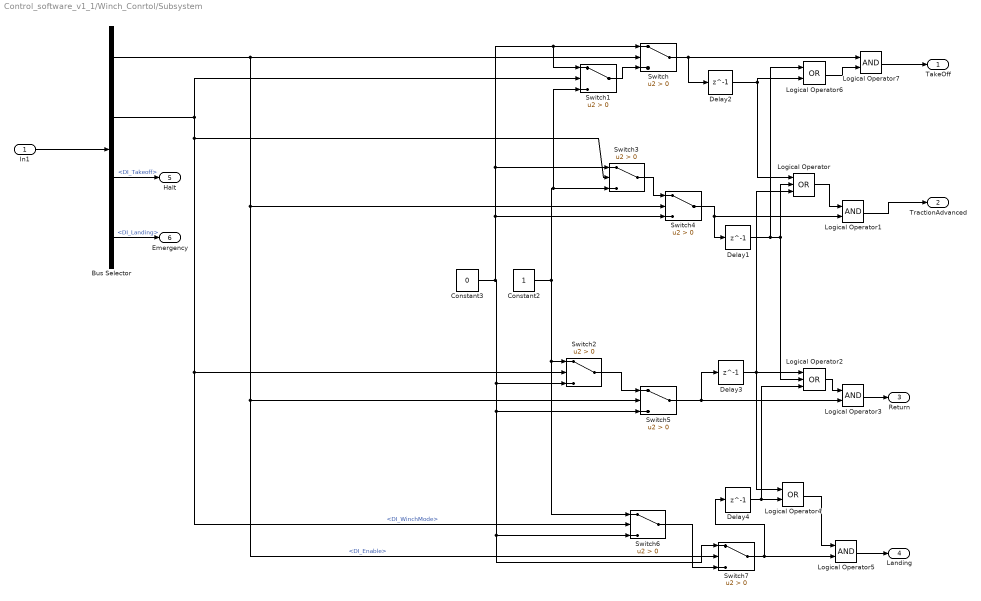
== system Control_software_v1_1/Winch_Conrtol/Subsystem ==
  In1 : Inport
  Bus Selector : BusSelector  OutputSignals=DgInputs.DI_Enable,DgInputs.DI_WinchMode,DgInputs.DI_Takeoff,DgInputs.DI_Landing
  Constant2 : Constant
  Constant3 : Constant  Value=0
  Delay{1..4} (4 alike) : Delay  DelayLength=1  InitialCondition=0
  Logical Operator : Logic  Operator=OR  Inputs=3  AllPortsSameDT=off  OutDataTypeStr=boolean
  Logical Operator{1,3,5,7} (4 alike) : Logic  AllPortsSameDT=off  OutDataTypeStr=boolean
  Logical Operator2 : Logic  Operator=OR  Inputs=3  AllPortsSameDT=off  OutDataTypeStr=boolean
  Logical Operator4 : Logic  Operator=OR  AllPortsSameDT=off  OutDataTypeStr=boolean
  Logical Operator6 : Logic  Operator=OR  AllPortsSameDT=off  OutDataTypeStr=boolean
  Switch{,1..7} (8 alike) : Switch  Criteria=u2 > Threshold
  TakeOff : Outport
  TractionAdvanced : Outport  Port=2
  Return : Outport  Port=3
  Landing : Outport  Port=4
  Halt : Outport  Port=5
  Emergency : Outport  Port=6
  wires:
  Switch3/1 -> Switch4/1
  Switch7/1 -> Delay4/1, Logical Operator5/2
  Delay3/1 -> Logical Operator4/1, Logical Operator/3, Logical Operator2/1
  Switch1/1 -> Switch/3
  Constant3/1 -> Switch4/3, Switch/1, Switch1/1, Switch3/1, Switch5/3, Switch6/3, Switch7/1, Switch2/3
  Bus Selector/2 -> Switch1/2, Switch3/2, Switch2/2, Switch6/2  "<DI_WinchMode>"
  Bus Selector/1 -> Switch/2, Switch7/2, Switch5/2, Switch4/2  "<DI_Enable>"
  Switch6/1 -> Switch7/3
  Switch/1 -> Logical Operator7/1, Delay2/1
  Logical Operator3/1 -> Return/1
  Delay4/1 -> Logical Operator2/3, Logical Operator4/2
  Logical Operator2/1 -> Logical Operator3/1
  Constant2/1 -> Switch6/1, Switch2/1, Switch1/3, Switch3/3
  In1/1 -> Bus Selector/1
  Logical Operator1/1 -> TractionAdvanced/1
  Switch4/1 -> Logical Operator1/2, Delay1/1
  Delay1/1 -> Logical Operator/2, Logical Operator2/2, Logical Operator6/1
  Logical Operator4/1 -> Logical Operator5/1
  Switch2/1 -> Switch5/1
  Delay2/1 -> Logical Operator/1, Logical Operator6/2
  Switch5/1 -> Logical Operator3/2, Delay3/1
  Logical Operator/1 -> Logical Operator1/1
  Logical Operator5/1 -> Landing/1
  Logical Operator6/1 -> Logical Operator7/2
  Logical Operator7/1 -> TakeOff/1
  Bus Selector/4 -> Emergency/1  "<DI_Landing>"
  Bus Selector/3 -> Halt/1  "<DI_Takeoff>"

== system Control_software_v1_1/Winch_Conrtol/damper ==
  SollWert : Inport
  Beschleunigung : Constant  Value=0.0025  SampleTime=0.001
  Compare To Zero : simulink/Logic and Bit Operations/Compare To Zero  relop=>  OutDataTypeStr=boolean
  Compare To Zero1 : simulink/Logic and Bit Operations/Compare To Zero  relop=<  OutDataTypeStr=boolean
  Constant1 : Constant  Value=0  SampleTime=0.001
  Delay : Delay  DelayLength=1  InitialCondition=0
  Delay1 : Delay  DelayLength=1  InitialCondition=0
  Gain : Gain  Gain=-1
  Sum : Sum  Inputs=|+-
  Sum1 : Sum  Inputs=|++
  Switch : Switch  Criteria=u2 > Threshold
  Switch1 : Switch  Criteria=u2 > Threshold
  Out1 : Outport
  wires:
  Sum/1 -> Compare To Zero1/1, Compare To Zero/1
  Compare To Zero/1 -> Switch/2
  Constant1/1 -> Switch/3
  Compare To Zero1/1 -> Switch1/2
  Switch/1 -> Switch1/3
  Gain/1 -> Switch1/1
  SollWert/1 -> Sum/1
  Switch1/1 -> Sum1/1
  Sum1/1 -> Delay/1, Delay1/1, Out1/1
  Delay/1 -> Sum/2
  Delay1/1 -> Sum1/2
  Beschleunigung/1 -> Switch/1, Gain/1

== system Control_software_v1_1/Input conditioning and estimators/Subsystem1/Subsystem ==
  AI_mot_winch_pos : Inport
  Constant : Constant  Value=WinchVoltMax
  Constant1 : Constant  Value=WinchTravelMin_m/WinchDrumRad
  Discrete Transfer Fcn1 : DiscreteTransferFcn  Numerator=WinchPosFiltNum  Denominator=WinchPosFiltDen
  Gain : Gain  Gain=WinchMotPosAIgain
  Sum : Sum  Inputs=++|
  Sum1 : Sum  Inputs=++|
  CI_WinchPos : Outport
  wires:
  AI_mot_winch_pos/1 -> Sum/2
  Discrete Transfer Fcn1/1 -> CI_WinchPos/1  "CI_WinchPos"
  Constant/1 -> Sum/1
  Gain/1 -> Sum1/2
  Sum/1 -> Gain/1
  Constant1/1 -> Sum1/1
  Sum1/1 -> Discrete Transfer Fcn1/1

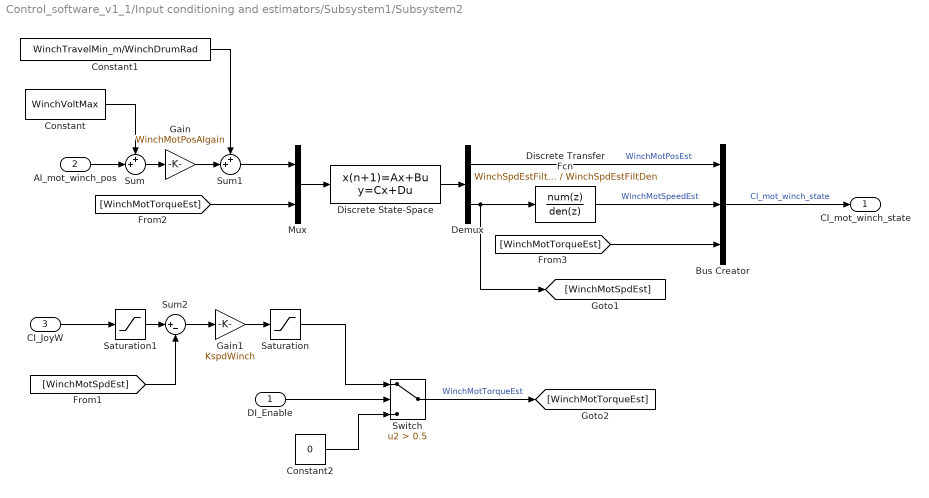
== system Control_software_v1_1/Input conditioning and estimators/Subsystem1/Subsystem2 ==
  DI_Enable : Inport
  AI_mot_winch_pos : Inport  Port=2
  CI_JoyW : Inport  Port=3
  Bus Creator : BusCreator  Inputs=3
  Constant : Constant  Value=WinchVoltMax
  Constant1 : Constant  Value=WinchTravelMin_m/WinchDrumRad
  Constant2 : Constant  Value=0
  Demux : Demux  Outputs=2
  Discrete Transfer Fcn : DiscreteTransferFcn  Numerator=WinchSpdEstFiltNum  Denominator=WinchSpdEstFiltDen
  Discrete State-Space : DiscreteStateSpace  A=Afilt_Winch  B=Bfilt_Winch  C=Cfilt_Winch  D=Dfilt_Winch  X0=x0_Winch  SampleTime=-1
  Gain : Gain  Gain=WinchMotPosAIgain
  Gain1 : Gain  Gain=KspdWinch
  Mux : Mux  Inputs=2
  Saturation : Saturate  UpperLimit=WinchMotTorqueMax  LowerLimit=-WinchMotTorqueMax
  Saturation1 : Saturate  UpperLimit=WinchRefSpdSup  LowerLimit=-WinchRefSpdSup
  Sum : Sum  Inputs=++|
  Sum1 : Sum  Inputs=++|
  Sum2 : Sum  Inputs=|+-
  Switch : Switch  Criteria=u2 > Threshold  Threshold=0.5
  CI_mot_winch_state : Outport
  wires:
  Bus Creator/1 -> CI_mot_winch_state/1  "CI_mot_winch_state"
  Demux/1 -> Bus Creator/1  "WinchMotPosEst"
  [WinchMotTorqueEst] -> Mux/2
  Sum1/1 -> Mux/1
  Discrete State-Space/1 -> Demux/1
  Mux/1 -> Discrete State-Space/1
  CI_JoyW/1 -> Saturation1/1
  AI_mot_winch_pos/1 -> Sum/2
  Constant/1 -> Sum/1
  Sum/1 -> Gain/1
  Constant1/1 -> Sum1/1
  Gain/1 -> Sum1/2
  Discrete Transfer Fcn/1 -> Bus Creator/2  "WinchMotSpeedEst"
  Demux/2 -> [WinchMotSpdEst], Discrete Transfer Fcn/1
  [WinchMotSpdEst] -> Sum2/2
  Sum2/1 -> Gain1/1
  Gain1/1 -> Saturation/1
  [WinchMotTorqueEst] -> Bus Creator/3
  DI_Enable/1 -> Switch/2
  Constant2/1 -> Switch/3
  Saturation1/1 -> Sum2/1
  Switch/1 -> [WinchMotTorqueEst]  "WinchMotTorqueEst"
  Saturation/1 -> Switch/1

== system Control_software_v1_1/Inputs/RS232_read/Compass_read ==
  ASCII_IMU : Inport
  Embedded MATLAB Function : MATLAB Function  TreatAsAtomicUnit=on
  FIFO ASCII read 1 : xpcseriallib/FIFO ASCII read   header={'$C'}  term=[42]  hold=Hold last output if no new data  enable=off  maxsize=40  outputtype=8 bit uint null terminated  sampletime=Ts_1s
      settings: SourceProductName=Simulink Real-Time  SourceProductBaseCode=XP
  Rate Transition4 : RateTransition  OutPortSampleTime=Ts_1s
  GU_Yaw : Outport
  wires:
  Embedded MATLAB Function/1(GU_Yaw) -> GU_Yaw/1  "GU_Yaw"
  FIFO ASCII read 1/1 -> Embedded MATLAB Function/1(in)
  ASCII_IMU/1 -> Rate Transition4/1
  Rate Transition4/1 -> FIFO ASCII read 1/1

== system Control_software_v1_1/Inputs/RS232_read/GPS_read ==
  ASCII_IMU : Inport
  Bus Creator : BusCreator  Inputs=4
  Embedded MATLAB Function : MATLAB Function  TreatAsAtomicUnit=on
  FIFO ASCII read 1 : xpcseriallib/FIFO ASCII read   header={'$GPGGA'}  term=[13 10]  hold=Hold last output if no new data  enable=off  maxsize=90  outputtype=8 bit uint null terminated  sampletime=Ts_1s
      settings: SourceProductName=Simulink Real-Time  SourceProductBaseCode=XP
  Rate Transition4 : RateTransition  OutPortSampleTime=Ts_1s
  GU_pos_data : Outport
  wires:
  Rate Transition4/1 -> FIFO ASCII read 1/1
  ASCII_IMU/1 -> Rate Transition4/1
  FIFO ASCII read 1/1 -> Embedded MATLAB Function/1(in)
  Embedded MATLAB Function/1(GU_Lat) -> Bus Creator/1  "GU_Lat"
  Embedded MATLAB Function/2(GU_Lon) -> Bus Creator/2  "GU_Lon"
  Embedded MATLAB Function/3(GU_h) -> Bus Creator/3  "GU_h"
  Embedded MATLAB Function/4(Geo_GU_h) -> Bus Creator/4  "Geo_Gu_h"
  Bus Creator/1 -> GU_pos_data/1  "GU_pos_data"

== system Control_software_v1_1/Inputs/RS232_read/IMU_read ==
  ASCII_IMU : Inport
  Bus Creator : BusCreator  Inputs=2
  Data_Check_CRC : Subsystem
  Data_validation : Subsystem
  "FIFO ASCII read " : xpcseriallib/FIFO ASCII read   header={[char(2),char(144),char(0),char(140)]}  term=[char(3) char(255)]  hold=Zero output if no new data  enable=off  maxsize=1024  outputtype=8 bit uint null terminated  sampletime=Ts_20ms
      settings: SourceProductName=Simulink Real-Time  SourceProductBaseCode=XP
  IMU_data_convert : Subsystem
  Rate Transition4 : RateTransition  OutPortSampleTime=Ts_20ms
  Selector : Selector  InputPortWidth=1025  IndexOptions=Index vector (dialog)  Indices=[2:146]  OutputSizes=162
  IMU_data_valid : Outport
  wires:
  "FIFO ASCII read "/1 -> Selector/1
  IMU_data_convert/1(IMU_data) -> [IMU_data]
  [IMU_data] -> Data_validation/1(IMU_data)
  Data_Check_CRC/1(Enable) -> Data_validation/Enable, Bus Creator/1
  Data_validation/1(IMU_data_valid) -> Bus Creator/2
  Selector/1 -> IMU_data_convert/1(ASCII_IMU), Data_Check_CRC/1(ASCII_IMU_crc)
  ASCII_IMU/1 -> Rate Transition4/1
  Rate Transition4/1 -> "FIFO ASCII read "/1
  Bus Creator/1 -> IMU_data_valid/1  "IMU_data_valid"

== system Control_software_v1_1/Winch_Conrtol/Joystick Regelung1/Joystick-Steuerung ==
  Joystick-Wert : Inport
  WinchSoll : Inport  Port=2
  Beschleunigung : Constant  Value=0.00125  SampleTime=0.001
  Gain : Gain  Gain=-1
  Relational Operator : RelationalOperator  OutDataTypeStr=boolean  RndMeth=Simplest
  Relational Operator1 : RelationalOperator  Operator=<  OutDataTypeStr=boolean  RndMeth=Simplest
  Sum : Sum  Inputs=|++
  Sum1 : Sum  Inputs=|++
  Switch : Switch  Criteria=u2 > Threshold
  Switch1 : Switch  Criteria=u2 > Threshold
  obere Grenze : Constant  SampleTime=0.001
  untere Grenze : Constant  Value=-1  SampleTime=0.001
  Out1 : Outport
  wires:
  Joystick-Wert/1 -> Relational Operator/1, Relational Operator1/1
  obere Grenze/1 -> Relational Operator/2
  Relational Operator/1 -> Switch/2
  untere Grenze/1 -> Relational Operator1/2
  Switch/1 -> Switch1/3
  Relational Operator1/1 -> Switch1/2
  Switch1/1 -> Out1/1
  WinchSoll/1 -> Sum1/2, Switch/3, Sum/2
  Beschleunigung/1 -> Gain/1, Sum/1
  Sum/1 -> Switch/1
  Gain/1 -> Sum1/1
  Sum1/1 -> Switch1/1

== system Control_software_v1_1/Winch_Conrtol/Joystick Regelung1/damper ==
  SollWert : Inport
  Beschleunigung : Constant  Value=0.00125  SampleTime=0.001
  Compare To Zero : simulink/Logic and Bit Operations/Compare To Zero  relop=>  OutDataTypeStr=boolean
  Compare To Zero1 : simulink/Logic and Bit Operations/Compare To Zero  relop=<  OutDataTypeStr=boolean
  Constant1 : Constant  Value=0  SampleTime=0.001
  Delay : Delay  DelayLength=1  InitialCondition=0
  Delay1 : Delay  DelayLength=1  InitialCondition=0
  Gain : Gain  Gain=-1
  Sum : Sum  Inputs=|+-
  Sum1 : Sum  Inputs=|++
  Switch : Switch  Criteria=u2 > Threshold
  Switch1 : Switch  Criteria=u2 > Threshold
  Out1 : Outport
  wires:
  Sum/1 -> Compare To Zero1/1, Compare To Zero/1
  Compare To Zero/1 -> Switch/2
  Constant1/1 -> Switch/3
  Compare To Zero1/1 -> Switch1/2
  Switch/1 -> Switch1/3
  Gain/1 -> Switch1/1
  SollWert/1 -> Sum/1
  Switch1/1 -> Sum1/1
  Sum1/1 -> Delay/1, Delay1/1, Out1/1
  Delay/1 -> Sum/2
  Delay1/1 -> Sum1/2
  Beschleunigung/1 -> Switch/1, Gain/1

== system Control_software_v1_1/Inputs/RS232_read/IMU_read/Data_Check_CRC ==
  ASCII_IMU_crc : Inport
  Demux : Demux  Outputs=[143 2]
  Embedded MATLAB Function : MATLAB Function  TreatAsAtomicUnit=on
  Enable : Outport
  wires:
  Demux/2 -> Embedded MATLAB Function/2(crc_in)
  Embedded MATLAB Function/1(CRC_valid) -> Enable/1
  ASCII_IMU_crc/1 -> Demux/1
  Demux/1 -> Embedded MATLAB Function/1(pBuffer)

== system Control_software_v1_1/Inputs/RS232_read/IMU_read/Data_validation ==
  IMU_data : Inport
  Enable : EnablePort
  IMU_data_valid : Outport
  wires:
  IMU_data/1 -> IMU_data_valid/1

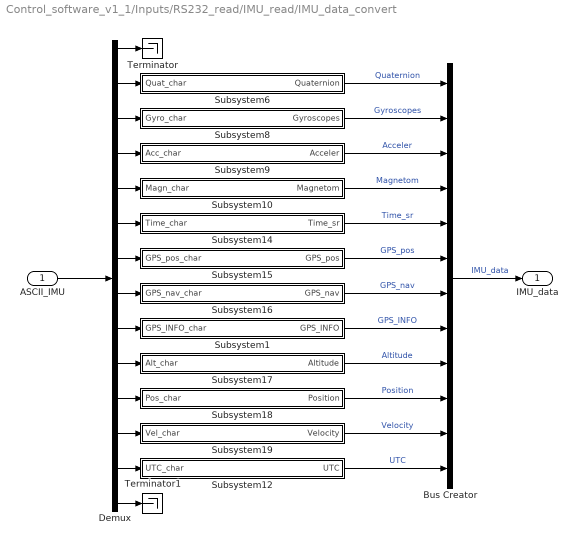
== system Control_software_v1_1/Inputs/RS232_read/IMU_read/IMU_data_convert ==
  ASCII_IMU : Inport
  Bus Creator : BusCreator  Inputs=12
  Demux : Demux  Outputs=[3 16 12 12 12 4 12 16 6 4 24 12 10 2]
  Subsystem1 : Subsystem
  Subsystem10 : Subsystem
  Subsystem12 : Subsystem
  Subsystem14 : Subsystem
  Subsystem15 : Subsystem
  Subsystem16 : Subsystem
  Subsystem17 : Subsystem
  Subsystem18 : Subsystem
  Subsystem19 : Subsystem
  Subsystem6 : Subsystem
  Subsystem8 : Subsystem
  Subsystem9 : Subsystem
  Terminator : Terminator
  Terminator1 : Terminator
  IMU_data : Outport
  wires:
  Bus Creator/1 -> IMU_data/1  "IMU_data"
  ASCII_IMU/1 -> Demux/1
  Demux/1 -> Terminator/1
  Demux/2 -> Subsystem6/1(Quat_char)
  Demux/3 -> Subsystem8/1(Gyro_char)
  Demux/4 -> Subsystem9/1(Acc_char)
  Demux/5 -> Subsystem10/1(Magn_char)
  Demux/6 -> Subsystem14/1(Time_char)
  Demux/14 -> Terminator1/1
  Subsystem6/1(Quaternion) -> Bus Creator/1  "Quaternion"
  Subsystem8/1(Gyroscopes) -> Bus Creator/2  "Gyroscopes"
  Subsystem9/1(Acceler) -> Bus Creator/3  "Acceler"
  Subsystem10/1(Magnetom) -> Bus Creator/4  "Magnetom"
  Subsystem14/1(Time_sr) -> Bus Creator/5  "Time_sr"
  Demux/7 -> Subsystem15/1(GPS_pos_char)
  Demux/8 -> Subsystem16/1(GPS_nav_char)
  Demux/9 -> Subsystem1/1(GPS_INFO_char)
  Demux/10 -> Subsystem17/1(Alt_char)
  Demux/11 -> Subsystem18/1(Pos_char)
  Demux/12 -> Subsystem19/1(Vel_char)
  Demux/13 -> Subsystem12/1(UTC_char)
  Subsystem15/1(GPS_pos) -> Bus Creator/6  "GPS_pos"
  Subsystem16/1(GPS_nav) -> Bus Creator/7  "GPS_nav"
  Subsystem1/1(GPS_INFO) -> Bus Creator/8  "GPS_INFO"
  Subsystem17/1(Altitude) -> Bus Creator/9  "Altitude"
  Subsystem18/1(Position) -> Bus Creator/10  "Position"
  Subsystem19/1(Velocity) -> Bus Creator/11  "Velocity"
  Subsystem12/1(UTC) -> Bus Creator/12  "UTC"

== system Control_software_v1_1/Inputs/RS232_read/IMU_read/IMU_data_convert/Subsystem1 ==
  GPS_INFO_char : Inport
  Bus Creator : BusCreator  Inputs=3
  Demux1 : Demux  Outputs=[4 1 1]
  Embedded MATLAB Function : MATLAB Function  TreatAsAtomicUnit=on
  Embedded MATLAB Function1 : MATLAB Function  TreatAsAtomicUnit=on
  Embedded MATLAB Function2 : MATLAB Function  TreatAsAtomicUnit=on
  GPS_INFO : Outport
  wires:
  GPS_INFO_char/1 -> Demux1/1
  Demux1/1 -> Embedded MATLAB Function/1(in)
  Embedded MATLAB Function/1(uint32_out) -> Bus Creator/1  "time"
  Demux1/2 -> Embedded MATLAB Function1/1(in)
  Demux1/3 -> Embedded MATLAB Function2/1(in)
  Embedded MATLAB Function1/1(uint8_out) -> Bus Creator/2  "GPSFlags"
  Embedded MATLAB Function2/1(uint8_out) -> Bus Creator/3  "NbSat"
  Bus Creator/1 -> GPS_INFO/1  "GPS_nav"

== system Control_software_v1_1/Inputs/RS232_read/IMU_read/IMU_data_convert/Subsystem10 ==
  Magn_char : Inport
  Bus Creator : BusCreator  Inputs=3
  Demux1 : Demux  Outputs=[4 4 4]
  Embedded MATLAB Function : MATLAB Function  TreatAsAtomicUnit=on
  Embedded MATLAB Function1 : MATLAB Function  TreatAsAtomicUnit=on
  Embedded MATLAB Function3 : MATLAB Function  TreatAsAtomicUnit=on
  Magnetom : Outport
  wires:
  Magn_char/1 -> Demux1/1
  Demux1/1 -> Embedded MATLAB Function/1(in)
  Demux1/2 -> Embedded MATLAB Function1/1(in)
  Demux1/3 -> Embedded MATLAB Function3/1(in)
  Embedded MATLAB Function/1(sing_out) -> Bus Creator/1  "Mx"
  Embedded MATLAB Function1/1(sing_out) -> Bus Creator/2  "My"
  Embedded MATLAB Function3/1(sing_out) -> Bus Creator/3  "Mz"
  Bus Creator/1 -> Magnetom/1  "Magnetom"

== system Control_software_v1_1/Inputs/RS232_read/IMU_read/IMU_data_convert/Subsystem12 ==
  UTC_char : Inport
  Bus Creator : BusCreator  Inputs=7
  Demux1 : Demux  Outputs=[1 1 1 1 1 1 4]
  Embedded MATLAB Function : MATLAB Function  TreatAsAtomicUnit=on
  Embedded MATLAB Function1 : MATLAB Function  TreatAsAtomicUnit=on
  Embedded MATLAB Function2 : MATLAB Function  TreatAsAtomicUnit=on
  Embedded MATLAB Function3 : MATLAB Function  TreatAsAtomicUnit=on
  Embedded MATLAB Function4 : MATLAB Function  TreatAsAtomicUnit=on
  Embedded MATLAB Function5 : MATLAB Function  TreatAsAtomicUnit=on
  Embedded MATLAB Function6 : MATLAB Function  TreatAsAtomicUnit=on
  UTC : Outport
  wires:
  UTC_char/1 -> Demux1/1
  Bus Creator/1 -> UTC/1  "UTC"
  Demux1/1 -> Embedded MATLAB Function/1(in)
  Demux1/2 -> Embedded MATLAB Function2/1(in)
  Demux1/3 -> Embedded MATLAB Function3/1(in)
  Demux1/4 -> Embedded MATLAB Function4/1(in)
  Demux1/5 -> Embedded MATLAB Function5/1(in)
  Demux1/6 -> Embedded MATLAB Function6/1(in)
  Demux1/7 -> Embedded MATLAB Function1/1(in)
  Embedded MATLAB Function/1(uint8_out) -> Bus Creator/1  "year"
  Embedded MATLAB Function2/1(uint8_out) -> Bus Creator/2  "month"
  Embedded MATLAB Function3/1(uint8_out) -> Bus Creator/3  "day"
  Embedded MATLAB Function4/1(uint8_out) -> Bus Creator/4  "hour"
  Embedded MATLAB Function5/1(uint8_out) -> Bus Creator/5  "min"
  Embedded MATLAB Function6/1(uint8_out) -> Bus Creator/6  "sec"
  Embedded MATLAB Function1/1(uint32_out) -> Bus Creator/7  "nanoseconds"

== system Control_software_v1_1/Inputs/RS232_read/IMU_read/IMU_data_convert/Subsystem14 ==
  Time_char : Inport
  Embedded MATLAB Function : MATLAB Function  TreatAsAtomicUnit=on
  Time_sr : Outport
  wires:
  Time_char/1 -> Embedded MATLAB Function/1(in)
  Embedded MATLAB Function/1(uint32_out) -> Time_sr/1  "Time_sr"

== system Control_software_v1_1/Inputs/RS232_read/IMU_read/IMU_data_convert/Subsystem15 ==
  GPS_pos_char : Inport
  Bus Creator : BusCreator  Inputs=3
  Demux1 : Demux  Outputs=[4 4 4]
  Embedded MATLAB Function1 : MATLAB Function  TreatAsAtomicUnit=on
  Embedded MATLAB Function2 : MATLAB Function  TreatAsAtomicUnit=on
  Embedded MATLAB Function3 : MATLAB Function  TreatAsAtomicUnit=on
  GPS_pos : Outport
  wires:
  GPS_pos_char/1 -> Demux1/1
  Bus Creator/1 -> GPS_pos/1  "GPS_pos"
  Embedded MATLAB Function2/1(int32_out) -> Bus Creator/3  "height"
  Embedded MATLAB Function1/1(int32_out) -> Bus Creator/2  "longitude"
  Embedded MATLAB Function3/1(int32_out) -> Bus Creator/1  "latitude"
  Demux1/3 -> Embedded MATLAB Function2/1(in)
  Demux1/2 -> Embedded MATLAB Function1/1(in)
  Demux1/1 -> Embedded MATLAB Function3/1(in)

== system Control_software_v1_1/Inputs/RS232_read/IMU_read/IMU_data_convert/Subsystem16 ==
  GPS_nav_char : Inport
  Bus Creator : BusCreator  Inputs=4
  Demux1 : Demux  Outputs=[4 4 4 4]
  Embedded MATLAB Function1 : MATLAB Function  TreatAsAtomicUnit=on
  Embedded MATLAB Function2 : MATLAB Function  TreatAsAtomicUnit=on
  Embedded MATLAB Function3 : MATLAB Function  TreatAsAtomicUnit=on
  Embedded MATLAB Function4 : MATLAB Function  TreatAsAtomicUnit=on
  GPS_nav : Outport
  wires:
  Demux1/1 -> Embedded MATLAB Function2/1(in)
  Demux1/2 -> Embedded MATLAB Function1/1(in)
  Demux1/3 -> Embedded MATLAB Function3/1(in)
  Embedded MATLAB Function2/1(int32_out) -> Bus Creator/1  "v_north"
  Embedded MATLAB Function1/1(int32_out) -> Bus Creator/2  "v_east"
  Embedded MATLAB Function3/1(int32_out) -> Bus Creator/3  "v_down"
  Bus Creator/1 -> GPS_nav/1  "GPS_nav"
  GPS_nav_char/1 -> Demux1/1
  Demux1/4 -> Embedded MATLAB Function4/1(in)
  Embedded MATLAB Function4/1(int32_out) -> Bus Creator/4  "heading"

== system Control_software_v1_1/Inputs/RS232_read/IMU_read/IMU_data_convert/Subsystem17 ==
  Alt_char : Inport
  Embedded MATLAB Function2 : MATLAB Function  TreatAsAtomicUnit=on
  Altitude : Outport
  wires:
  Alt_char/1 -> Embedded MATLAB Function2/1(in)
  Embedded MATLAB Function2/1(int32_out) -> Altitude/1  "Altitude"

== system Control_software_v1_1/Inputs/RS232_read/IMU_read/IMU_data_convert/Subsystem18 ==
  Pos_char : Inport
  Bus Creator : BusCreator  Inputs=3
  Demux1 : Demux  Outputs=[8 8 8]
  Embedded MATLAB Function : MATLAB Function  TreatAsAtomicUnit=on
  Embedded MATLAB Function1 : MATLAB Function  TreatAsAtomicUnit=on
  Embedded MATLAB Function2 : MATLAB Function  TreatAsAtomicUnit=on
  Position : Outport
  wires:
  Bus Creator/1 -> Position/1  "Position"
  Pos_char/1 -> Demux1/1
  Demux1/1 -> Embedded MATLAB Function/1(in)
  Demux1/2 -> Embedded MATLAB Function1/1(in)
  Demux1/3 -> Embedded MATLAB Function2/1(in)
  Embedded MATLAB Function2/1(double_out) -> Bus Creator/3  "height_filt"
  Embedded MATLAB Function1/1(double_out) -> Bus Creator/2  "long_filt"
  Embedded MATLAB Function/1(double_out) -> Bus Creator/1  "lat_filt"

== system Control_software_v1_1/Inputs/RS232_read/IMU_read/IMU_data_convert/Subsystem19 ==
  Vel_char : Inport
  Bus Creator : BusCreator  Inputs=3
  Demux1 : Demux  Outputs=[4 4 4]
  Embedded MATLAB Function : MATLAB Function  TreatAsAtomicUnit=on
  Embedded MATLAB Function1 : MATLAB Function  TreatAsAtomicUnit=on
  Embedded MATLAB Function3 : MATLAB Function  TreatAsAtomicUnit=on
  Velocity : Outport
  wires:
  Embedded MATLAB Function/1(sing_out) -> Bus Creator/1  "Vx"
  Embedded MATLAB Function1/1(sing_out) -> Bus Creator/2  "Vy"
  Embedded MATLAB Function3/1(sing_out) -> Bus Creator/3  "Vz"
  Demux1/3 -> Embedded MATLAB Function3/1(in)
  Demux1/2 -> Embedded MATLAB Function1/1(in)
  Demux1/1 -> Embedded MATLAB Function/1(in)
  Vel_char/1 -> Demux1/1
  Bus Creator/1 -> Velocity/1  "Velocity"
